simulink model "sim_double_pendulum"  (R2015a)
settings: Solver=ode45  StartTime=0.0  StopTime=10.0  RelTol=1e-3
values from neighbouring files (symbols this model uses):
  params = catstruct(params, sys.params_str)    [double_lqg.m]    (also in load_mechanism_params.m = params(1:13); load_params.m = [g, m0, b0,                m1, I1, b1, L1, L1_cg,           ; load_single_mechanism_params.m = params(1:8); load_single_params.m = [g, m0, b0,                m1, I1, b1, L1, L1_cg,           )
  sys = double_pendulum(Ts, ndelay)    [double_lqg.m]    (also in double_pendulum_mechanics.m = dynamic_model(sys); lin_pendulum.m = plant_behaviour(sys); load_double_sys.m; load_single_sys.m = single_pendulum())
libraries: aerolibutil x1
settings Model: Creator=BPeixoto  LastModifiedBy=BPeixoto

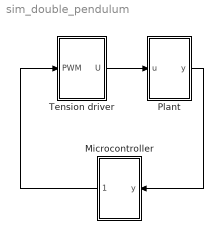
== system sim_double_pendulum ==
  Microcontroller : Subsystem
  Plant : Subsystem
  Tension driver : Subsystem
  wires:
  Tension driver/1(U) -> Plant/1(u)
  Plant/1(y) -> Microcontroller/1(y)
  Microcontroller/1(PWM) -> Tension driver/1(PWM)

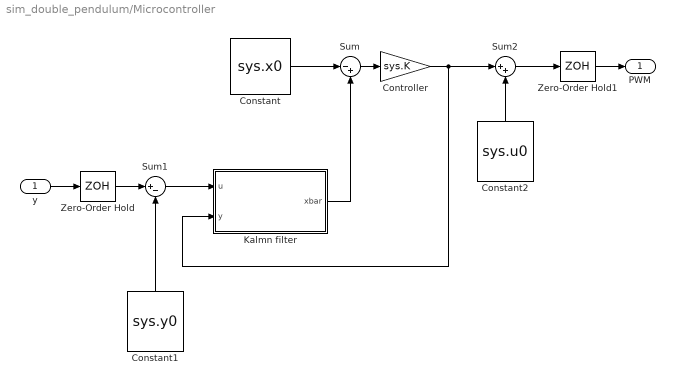
== system sim_double_pendulum/Microcontroller ==
  y : Inport
  Constant : Constant  Value=sys.x0
  Constant1 : Constant  Value=sys.y0
  Constant2 : Constant  Value=sys.u0
  Controller : Gain  Gain=sys.K
  Kalmn filter : MATLAB Function  TreatAsAtomicUnit=on
  Sum : Sum  Inputs=|-+
  Sum1 : Sum  Inputs=|+-
  Sum2 : Sum  Inputs=|++
  Zero-Order Hold : ZeroOrderHold
  Zero-Order Hold1 : ZeroOrderHold
  PWM : Outport
  wires:
  y/1 -> Zero-Order Hold/1
  Constant/1 -> Sum/1
  Sum/1 -> Controller/1
  Kalmn filter/1(xbar) -> Sum/2
  Sum1/1 -> Kalmn filter/1(u)
  Constant1/1 -> Sum1/2
  Zero-Order Hold/1 -> Sum1/1
  Zero-Order Hold1/1 -> PWM/1
  Controller/1 -> Sum2/1, Kalmn filter/2(y)
  Constant2/1 -> Sum2/2
  Sum2/1 -> Zero-Order Hold1/1

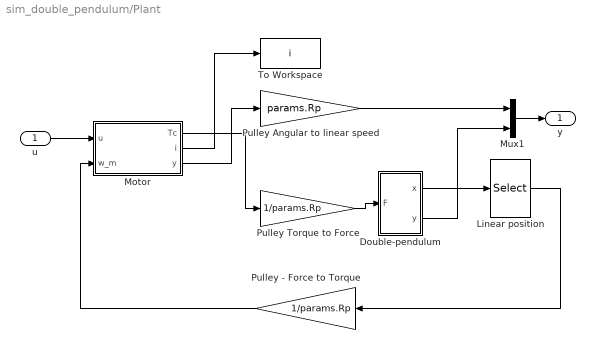
== system sim_double_pendulum/Plant ==
  u : Inport
  Double-pendulum : Subsystem
  Linear position : Selector  InputPortWidth=6  Indices=[4]
  Motor : MATLAB Function  TreatAsAtomicUnit=on
  Mux1 : Mux  Inputs=2
  Pulley Torque to Force : Gain  Gain=1/params.Rp
  Pulley Angular to linear speed : Gain  Gain=params.Rp
  Pulley - Force to Torque : Gain  Gain=1/params.Rp
  To Workspace : ToWorkspace  VariableName=i  SaveFormat=Timeseries  SampleTime=-1
  y : Outport
  wires:
  Pulley Torque to Force/1 -> Double-pendulum/1(F)
  Double-pendulum/2(y) -> Mux1/2
  Motor/1(Tc) -> Pulley Torque to Force/1
  Mux1/1 -> y/1
  u/1 -> Motor/1(u)
  Motor/3(y) -> Pulley Angular to linear speed/1
  Pulley Angular to linear speed/1 -> Mux1/1
  Double-pendulum/1(x) -> Linear position/1
  Linear position/1 -> Pulley - Force to Torque/1
  Pulley - Force to Torque/1 -> Motor/2(w_m)
  Motor/2(i) -> To Workspace/1

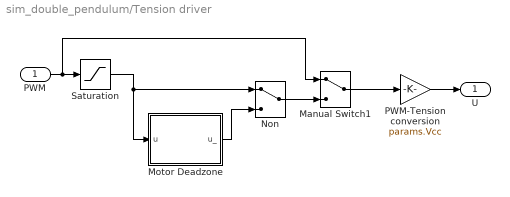
== system sim_double_pendulum/Tension driver ==
  PWM : Inport
  Manual Switch1 : ManualSwitch
  Motor Deadzone : MATLAB Function  TreatAsAtomicUnit=on
  Non : ManualSwitch
  PWM-Tension conversion : Gain  Gain=params.Vcc
  Saturation : Saturate  UpperLimit=1  LowerLimit=-1
  U : Outport
  wires:
  PWM/1 -> Manual Switch1/1, Saturation/1
  PWM-Tension conversion/1 -> U/1
  Saturation/1 -> Motor Deadzone/1(u), Non/1
  Motor Deadzone/1(u_) -> Non/2
  Non/1 -> Manual Switch1/2
  Manual Switch1/1 -> PWM-Tension conversion/1

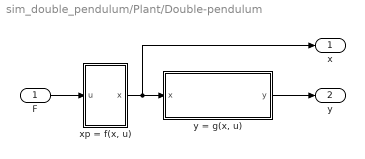
== system sim_double_pendulum/Plant/Double-pendulum ==
  F : Inport
  "xp = f(x, u)" : Subsystem
  "y = g(x, u)" : MATLAB Function  TreatAsAtomicUnit=on
  x : Outport
  y : Outport  Port=2
  wires:
  F/1 -> "xp = f(x, u)"/1(u)
  "y = g(x, u)"/1(y) -> y/1
  "xp = f(x, u)"/1(x) -> x/1, "y = g(x, u)"/1(x)

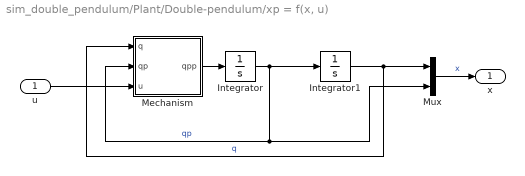
== system sim_double_pendulum/Plant/Double-pendulum/xp = f(x, u) ==
  u : Inport
  Integrator : Integrator
  Integrator1 : Integrator
  Mechanism : Subsystem
  Mux : Mux  Inputs=2
  x : Outport
  wires:
  Mux/1 -> x/1  "x"
  u/1 -> Mechanism/3(u)
  Integrator/1 -> Mux/2, Mechanism/2(qp), Integrator1/1  "qp"
  Mechanism/1(qpp) -> Integrator/1
  Integrator1/1 -> Mux/1, Mechanism/1(q)  "q"

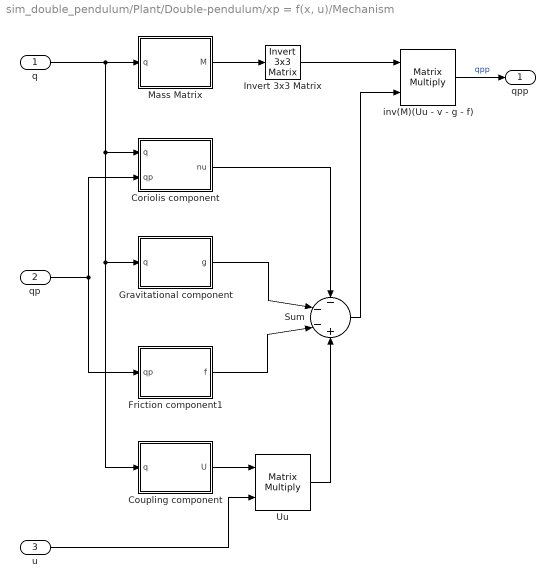
== system sim_double_pendulum/Plant/Double-pendulum/xp = f(x, u)/Mechanism ==
  q : Inport
  qp : Inport  Port=2
  u : Inport  Port=3
  Coriolis component : MATLAB Function  TreatAsAtomicUnit=on
  Coupling component : MATLAB Function  TreatAsAtomicUnit=on
  Friction component1 : MATLAB Function  TreatAsAtomicUnit=on
  Gravitational component : MATLAB Function  TreatAsAtomicUnit=on
  Invert 3x3 Matrix : aerolibutil/Invert  3x3 Matrix
  Mass Matrix : MATLAB Function  TreatAsAtomicUnit=on
  Sum : Sum  Inputs=-|-|-|+
  Uu : Product  Multiplication=Matrix(*)
  inv(M)(Uu - v - g - f) : Product  Multiplication=Matrix(*)
  qpp : Outport
  wires:
  Mass Matrix/1(M) -> Invert 3x3 Matrix/1
  Coriolis component/1(nu) -> Sum/1
  qp/1 -> Coriolis component/2(qp), Friction component1/1(qp)
  q/1 -> Coupling component/1(q), Gravitational component/1(q), Coriolis component/1(q), Mass Matrix/1(q)
  Gravitational component/1(g) -> Sum/2
  Friction component1/1(f) -> Sum/3
  Invert 3x3 Matrix/1 -> inv(M)(Uu - v - g - f)/1
  Sum/1 -> inv(M)(Uu - v - g - f)/2
  inv(M)(Uu - v - g - f)/1 -> qpp/1  "qpp"
  Coupling component/1(U) -> Uu/1
  u/1 -> Uu/2
  Uu/1 -> Sum/4

== matlab function sim_double_pendulum/Plant/Double-pendulum/xp = f(x, u)/Mechanism/Coriolis component ==
  data: q input; qp input; nu output; params parameter
function nu = corvec(q, qp, params)
    % Coriolis 'vector
    nu = zeros(3, 1);
    
    % Coupled mass matrix
    nu(1,1) = -params.m2*params.L2g*sin(q(1) + q(2)) + (qp(1) + qp(2)^2 - (params.m2*params.L1 + params.m1*params.L1g)*sin(q(1))*qp(1)^2);
    nu(2,2) = -params.m2*qp(2)*(2*qp(1) + qp(2))*params.L2g*params.L1*sin(q(2));
    nu(3,3) = params.m2*params.L2g*params.L1*sin(q(2));
end

== matlab function sim_double_pendulum/Plant/Double-pendulum/xp = f(x, u)/Mechanism/Mass Matrix ==
  data: q input; M output; params parameter
function M = mmatrix(q, params)
    % Mass matrix
    M = zeros(3, 3);
    
    % Coupled mass matrix
    M(1,1) = params.m0 + params.m1 + params.m2;
    M(2,2) = params.m2*params.L2g^2 + params.I2;
    M(3,3) = params.m1*params.L1g^2 + ...
             params.m2*(params.L1^2 + params.L2^2) +...
             params.I1 + 2*params.m2*params.L1*params.L2d*cos(q(2));
         
    M(1,2) = params.m2*params.L2g*cos(q(1) + q(2)) + ...
            (params.m2*params.L1 + params.l1g)*cos(q(1));
    M(1,3) = params.m2*params.L2g*cos(q(1) + q(2));
    M(2,3) = params.m2*params.L2g^2 + params.I2 + ...
             params.m2*params.L1*params.L2g*cos(q(2));
    
    M(2,1) = M(1,2);
    M(3,1) = M(1,3);
    M(3,2) = M(2,3);
end

== matlab function sim_double_pendulum/Plant/Double-pendulum/xp = f(x, u)/Mechanism/Gravitational component ==
  data: q input; g output; params parameter
function g = gvec(q, params)
    % Gravitational component
    g = zeros(3, 1);
    
    % Coupled mass matrix
    g(1,1) = 0;
    g(2,2) = params.m2*params.g*(params.L1*sin(q(1) + params.L2g*sin(q(1) + q(2))) + params.m1*params.L1*params.g*sin(q(1)));
    g(3,3) = params.m2*params.g*params.L2g*sin(q(1) + q(2));
end

== matlab function sim_double_pendulum/Plant/Double-pendulum/xp = f(x, u)/Mechanism/Friction component1 ==
  data: qp input; f output; params parameter
function f = fvec(qp, params)
    % Friction vector
    f = zeros(3, 1);
    
    % Coupled mass matrix
    f(1,1) = params.b0*qp(1);
    f(2,2) = params.b1*qp(1);
    f(3,3) = params.b2*qp(1);
end

== matlab function sim_double_pendulum/Plant/Double-pendulum/xp = f(x, u)/Mechanism/Coupling component ==
  data: q input; U output; params parameter
function U = Uvec(q, params)
    U = [1; 0; 0];
end

== matlab function sim_double_pendulum/Plant/Double-pendulum/y = g(x, u) ==
  data: x input; y output
function y = pendulum_output(x)
    y = [x(2); x(3)];
end

== matlab function sim_double_pendulum/Microcontroller/Kalmn filter ==
  data: u input; y input; xbar output; params parameter
function xbar = kalman_filter(u, y, params)
    % First assignemnt
    persistent M;
    persistent x_bar;
    
    if isempty(M)
        M = params.M0;
    end
    
    if isempty(x_bar)
        xbar = params.xbar0;
    end
    
    % Main matrices
    Phi = params.Phi;
    Gamma = params.Gamma;

    C = params.C;
    Psi = params.Psi;
    
    Rv = params.Rv;
    Rw = params.Rw;
    
    % Stationary Ricatti equation solution
    P = M - M*C'*(C*M*C' + Rv)*C*M;
    
    % Observer gain
    Lc = P*C'/Rv;
    
    % Time update
    x_hat = xbar + Lc*(y - C*x_bar);
    
    % Measurement update
    x_bar = Phi*x_hat + Gamma*u;
    
    % M update
    M = Phi*P*Phi' + Psi*Rw*Psi';
end

== matlab function sim_double_pendulum/Plant/Motor ==
  data: Tc output; i output; y output; u input; w_m input; params parameter
function [Tc, i, y] = motor(u, w_m, params)
    % Motor parameters
    % Simplifications: 
    %   Negligible pulley inertia and stator inductance
    R = params.R;
    Kt = params.Kt;
    Ke = params.Ke;
    bm = params.bm;
    
    % Exerted Torque
    Tc = (Kt/R)*(u - (R*bm/Kt + Ke)*w_m);
    i = (Tc + bm*w_m)   /Kt;
    y = w_m;

== matlab function sim_double_pendulum/Tension driver/Motor Deadzone ==
  data: u input; u_ output; params parameter
function u_ = deadzone(u, params)
    if(u > params.deadzone || u < -params.deadzone) 
        u_ = 0;
    else
        u_ = u;
    end
end
